simulink model "Test_Bit_Multiplexer_16_to_1_NAND"  (R2023a)
settings: Solver=ode45  StartTime=0.0  StopTime=len  RelTol=1e-3  EnableMultiTasking=on
libraries: simulink x2, Bit_Multiplexers_Lib x1
settings Model: Creator=N  LastModifiedBy=Jozko Mrkvicka
settings SolverCC: AlgebraicLoopSolver=TrustRegion
settings DataIOCC: SaveFormat=Array  ReturnWorkspaceOutputs=off
settings OptimizationCC: LifeSpan=inf
settings DebuggingCC: UnconnectedInputMsg=warning  UnconnectedOutputMsg=warning  UnconnectedLineMsg=warning  SFUnexpectedBacktrackingDiag=warning  SFNoUnconditionalDefaultTransitionDiag=warning  SFExecutionAtInitializationDiag=none  ArithmeticOperatorsInVariantConditions=warning
settings HardwareCC: ProdWordSize=32
settings SFSimCC: SimUseLocalCustomCode=off  CustomCodeUndefinedFunction=UseInterfaceOnly
settings RTWCC: RTWUseLocalCustomCode=off
settings CodeAppCC: StateflowObjectComments=on
settings GRTTargetCC: TargetLangStandard=C89/C90 (ANSI)
settings ConfigComp: CovMetricSettings=dw  CovSaveCumulativeToWorkspaceVar=on  CovSaveSingleToWorkspaceVar=on  CovExternalEMLEnable=off

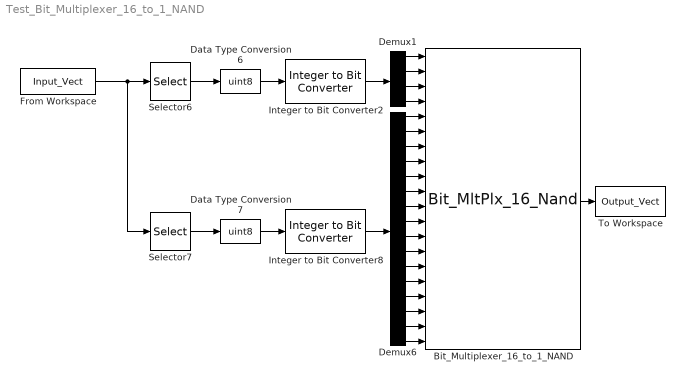
== system Test_Bit_Multiplexer_16_to_1_NAND ==
  Bit_Multiplexer_16_to_1_NAND : Bit_Multiplexers_Lib/Bit_MltPlx_16_Nand  SystemSampleTime=-1  VariantActivationTime=update diagram  Latency=0  AutoFrameSizeCalculation=off
  Data Type Conversion6 : DataTypeConversion  OutDataTypeStr=uint8  SaturateOnIntegerOverflow=off  RndMeth=Floor
  Data Type Conversion7 : DataTypeConversion  OutDataTypeStr=uint8  SaturateOnIntegerOverflow=off  RndMeth=Floor
  Demux1 : Demux
  Demux6 : Demux  Outputs=16
  From Workspace : FromWorkspace  VariableName=Input_Vect  SampleTime=1  Interpolate=off  ZeroCross=off  OutputAfterFinalValue=Holding final value
  Integer to Bit Converter2 : simulink/Logic and Bit Operations/Integer to Bit Converter  nbits=4  signedInputValues=Unsigned  bitOrder=MSB first  outDtype=boolean
      settings: LibrarySourceBlock=|
      | commutil2/Integer to Bit
      | Converter
  Integer to Bit Converter8 : simulink/Logic and Bit Operations/Integer to Bit Converter  nbits=16  signedInputValues=Unsigned  bitOrder=MSB first  outDtype=uint8
      settings: LibrarySourceBlock=|
      | commutil2/Integer to Bit
      | Converter
  Selector6 : Selector  IndexMode=Zero-based  InputPortWidth=2  SampleTime=1  IndexOptions=Index vector (dialog)  Indices=0  OutputSizes=1
  Selector7 : Selector  IndexMode=Zero-based  InputPortWidth=2  IndexOptions=Index vector (dialog)  Indices=1  OutputSizes=1
  To Workspace : ToWorkspace  VariableName=Output_Vect  SampleTime=1
  wires:
  Integer to Bit Converter8/1 -> Demux6/1
  Demux1/1 -> Bit_Multiplexer_16_to_1_NAND/1
  Demux1/2 -> Bit_Multiplexer_16_to_1_NAND/2
  Demux1/3 -> Bit_Multiplexer_16_to_1_NAND/3
  Demux1/4 -> Bit_Multiplexer_16_to_1_NAND/4
  Integer to Bit Converter2/1 -> Demux1/1
  Demux6/1 -> Bit_Multiplexer_16_to_1_NAND/5
  Demux6/2 -> Bit_Multiplexer_16_to_1_NAND/6
  Demux6/3 -> Bit_Multiplexer_16_to_1_NAND/7
  Demux6/4 -> Bit_Multiplexer_16_to_1_NAND/8
  Demux6/5 -> Bit_Multiplexer_16_to_1_NAND/9
  Demux6/6 -> Bit_Multiplexer_16_to_1_NAND/10
  Demux6/7 -> Bit_Multiplexer_16_to_1_NAND/11
  Demux6/8 -> Bit_Multiplexer_16_to_1_NAND/12
  Demux6/9 -> Bit_Multiplexer_16_to_1_NAND/13
  Demux6/10 -> Bit_Multiplexer_16_to_1_NAND/14
  Demux6/11 -> Bit_Multiplexer_16_to_1_NAND/15
  Demux6/12 -> Bit_Multiplexer_16_to_1_NAND/16
  Demux6/13 -> Bit_Multiplexer_16_to_1_NAND/17
  Demux6/14 -> Bit_Multiplexer_16_to_1_NAND/18
  Demux6/15 -> Bit_Multiplexer_16_to_1_NAND/19
  Demux6/16 -> Bit_Multiplexer_16_to_1_NAND/20
  From Workspace/1 -> Selector7/1, Selector6/1
  Selector6/1 -> Data Type Conversion6/1
  Selector7/1 -> Data Type Conversion7/1
  Data Type Conversion6/1 -> Integer to Bit Converter2/1
  Data Type Conversion7/1 -> Integer to Bit Converter8/1
  Bit_Multiplexer_16_to_1_NAND/1 -> To Workspace/1
